simulink model "Example_RPI_Xroad_American.exec"  (Simulink 3.00)
settings: Solver=ode45  SolverMode=SingleTasking  StartTime=0.0  StopTime=10.0  RelTol=1e-3
libraries: execlib x7
settings Model: ExtModeTrigMode=normal  ExtModeArmWhenConnect=on  Creator=ojezek  LastModifiedBy=XPMUser

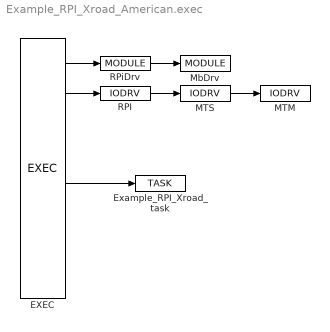
== system Example_RPI_Xroad_American.exec ==
  EXEC : execlib/EXEC  target=PC - Linux  tick=0.05  ntick0=2  ntick1=12  ntick2=15  ntick3=20  pri0=5  pri1=9  pri2=13  pri3=18
  Example_RPI_Xroad_task : execlib/TASK  factor=1  start=0  stop=1  stack=10240  MDLOPEN=off  bEdit=off
  MTM : execlib/IODRV  SystemSampleTime=-1  module=MbDrv  classname=MtmDrv  cfgname=MbDrvM.rio  factor=5  stack=10240  pri=3  bEdit=off  timer=off
  MTS : execlib/IODRV  SystemSampleTime=-1  module=MbDrv  classname=MtsDrv  cfgname=MbDrv.rio  factor=5  stack=10240  pri=3  bEdit=off  timer=off
  MbDrv : execlib/MODULE  SystemSampleTime=-1
  RPI : execlib/IODRV  module=RPiDrv  classname=RPiDrv  factor=1  stack=10240  pri=3  timer=off
  RPiDrv : execlib/MODULE
  wires:
  EXEC/1 -> RPiDrv/1
  EXEC/2 -> RPI/1
  EXEC/5 -> Example_RPI_Xroad_task/1
  MTS/1 -> MTM/1
  RPI/1 -> MTS/1
  RPiDrv/1 -> MbDrv/1
